simulink model "MPC"  (R2023a)
settings: Solver=VariableStepAuto  StartTime=0.0  StopTime=1000  RelTol=1e-3
undefined symbols (not defined in the file): A, B, C, D
libraries: mpclib x1
settings Model: Creator=vitor  LastModifiedBy=vitor

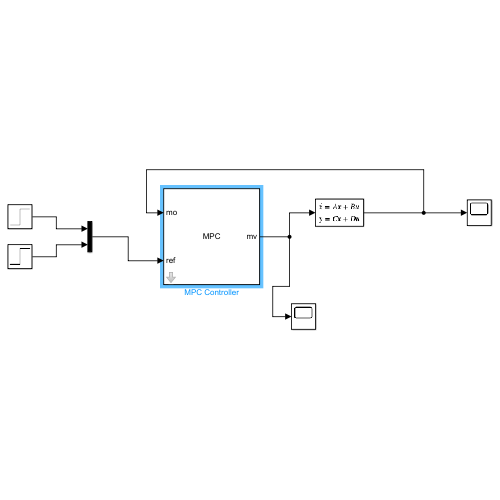
[thumbnail: Simulink's stored preview of the top-level diagram]
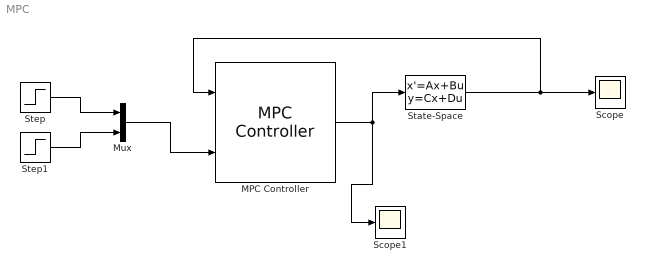
== system MPC ==
  MPC Controller : mpclib/MPC Controller  SCDEnableBlockLinearizationSpecification=on  mpcobj=mpc3  is_multiple=0  enable_value=0  return_u0=off  updateMPCinCallerWorkspace=on  md_inport=off  mv_inport=off  uref_inport=off  return_cost=off  return_mvseq=off  return_qpstatus=off  return_xseq=off  return_state=off  return_ovseq=off  state_inport=off  umin_inport=off  umax_inport=off  ymin_inport=off  ymax_inport=off  cc_inport=off  ywt_inport=off  uwt_inport=off  duwt_inport=off  rhoeps_inport=off  pm_inport=off  MaximumP=10  HorizonChoice=FixedHorizon  n_ts=1  n_p=10  n_mv=2  n_md=0  n_ud=0  n_mo=2  n_uo=0  BlockDataType=double  SampleTimeInherited=off  switch_inport=off
  Mux : Mux  Inputs=2
  Scope : Scope
  Scope1 : Scope
  State-Space : StateSpace  A=A  B=B  C=C  D=D  InitialCondition=0
  Step : Step  Time=30  SampleTime=0
  Step1 : Step  Time=500  SampleTime=0
  wires:
  MPC Controller/1 -> State-Space/1, Scope1/1
  State-Space/1 -> MPC Controller/1, Scope/1
  Step/1 -> Mux/1
  Step1/1 -> Mux/2
  Mux/1 -> MPC Controller/2
